simulink model "exp2_model"  (R2019b)
settings: Solver=FixedStepAuto  StartTime=0.0  StopTime=5  FixedStep=0.000001  RelTol=1e-3
values from neighbouring files (symbols this model uses):
  Io = 0    [exp2_script.m]
  Jeq = 1.16e-6+.5*0.068*.0248^2    (= 2.207136e-05)    [exp2_script.m]
  K = 1/(km+Rm*Io)    (= 19.9203187251)    [exp2_script.m]    (also in measured_data_plots.m = 14.5)
  km = 0.0502    [exp2_script.m]
  kt = 0.0502    [exp2_script.m]
  Ktd = -Rm/(kt*km+Rm*kt*Io)    (= -4206.28243996)    [exp2_script.m]
  Rm = 10.6    [exp2_script.m]
  Rm_measured = 1/ft.p1    [resistance_measurements.m]
  tau = Jeq*Rm/(kt*km+Rm*kt*Io)    (= 0.0928383739941)    [exp2_script.m]    (also in measured_data_plots.m = 0.09)
  tau_td = Jeq*Rm/(kt*km+Rm*kt*Io)    (= 0.0928383739941)    [exp2_script.m]
  wf = 1/0.1    (= 10)    [exp2_script.m]
undefined symbols (not defined in the file or in its folder): ki, kp
libraries: simulink x1, powerlib_meascontrol x1
settings Model: SimulationMode=accelerator  Creator=irex  LastModifiedBy=isaac
settings SolverCC: AlgebraicLoopSolver=LineSearch
settings SFSimCC: CustomCodeUndefinedFunction=UseInterfaceOnly

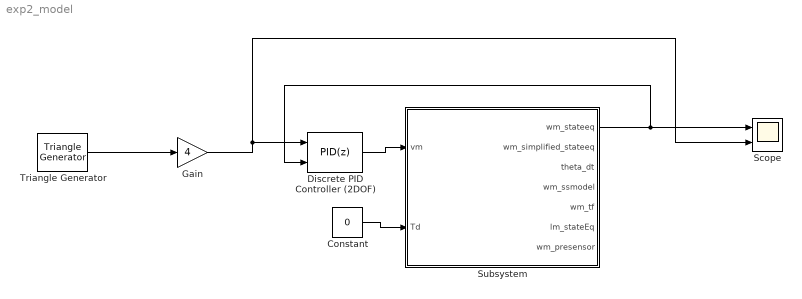
== system exp2_model ==
  Constant : Constant  Value=0
  Discrete PID Controller (2DOF) : simulink/Continuous/PID Controller (2DOF)  Controller=PID  Form=Parallel  TimeDomain=Discrete-time  SampleTime=-1  IntegratorMethod=Forward Euler  FilterMethod=Forward Euler  ControllerParametersSource=internal  P=kp  I=ki  D=0  UseFilter=on  N=100  b=1  c=1  TunerSelectOption=Transfer Function Based (PID Tuner App)  InitialConditionSource=internal  InitialConditionForIntegrator=0  InitialConditionForFilter=0  DifferentiatorICPrevScaledInput=0  ExternalReset=none  TrackingMode=off  Kt=1  LimitOutput=off  UpperSaturationLimit=inf  LowerSaturationLimit=-inf  LinearizeAsGain=off  AntiWindupMode=none  Kb=1  POutMin=[]  POutMax=[]  IOutMin=[]  IOutMax=[]  DOutMin=[]  DOutMax=[]  NOutMin=[]  NOutMax=[]  bOutMin=[]  bOutMax=[]  cOutMin=[]  cOutMax=[]  SumOutMin=[]  SumOutMax=[]  SaturationOutMin=[]  SaturationOutMax=[]  PParamMin=[]  PParamMax=[]  IParamMin=[]  IParamMax=[]  DParamMin=[]  DParamMax=[]  NParamMin=[]  NParamMax=[]  bParamMin=[]  bParamMax=[]  cParamMin=[]  cParamMax=[]  KbParamMin=[]  KbParamMax=[]  KtParamMin=[]  KtParamMax=[]  KbOutMin=[]  KbOutMax=[]  KtOutMin=[]  KtOutMax=[]  IntegratorOutMin=[]  IntegratorOutMax=[]  FilterOutMin=[]  FilterOutMax=[]  SumI1OutMin=[]  SumI1OutMax=[]  SumI2OutMin=[]  SumI2OutMax=[]  SumI3OutMin=[]  SumI3OutMax=[]  SumI4OutMin=[]  SumI4OutMax=[]  SumDOutMin=[]  SumDOutMax=[]  Sum1OutMin=[]  Sum1OutMax=[]  Sum2OutMin=[]  Sum2OutMax=[]  Sum3OutMin=[]  Sum3OutMax=[]  DifferentiatorOutMin=[]  DifferentiatorOutMax=[]  FilterDiffOutCoefMin=[]  FilterDiffOutCoefMax=[]  ReciprocalOutMin=[]  ReciprocalOutMax=[]  SumDenOutMin=[]  SumDenOutMax=[]  SumNumOutMin=[]  SumNumOutMax=[]  DivideOutMin=[]  DivideOutMax=[]  IntegratorContinuousStateAttributes=''  IntegratorStateMustResolveToSignalObject=off  IntegratorRTWStateStorageClass=Auto  FilterContinuousStateAttributes=''  FilterStateMustResolveToSignalObject=off  FilterRTWStateStorageClass=Auto  ParallelPVariant=InternalParameters  IdealPVariant=Disabled  IVariant=InternalParameters  DVariant=InternalParameters  bVariant=InternalParameters  cVariant=InternalParameters  IntegratorVariant=Discrete  SatVariant=Disabled  AWVariant=Passthrough  PCopyVariant=Disabled  TRVariant=Disabled  FdbkBlocksVariant=Forward  IdealPFdbkVariant=Disabled  SatFdbkVariant=Disabled  DerivativeFilterVariant=ForwardEulerFilter  NVariant=InternalParameters  NCopyVariant=Disabled  FilterICVariant=InternalICsFilter  IntegratorICVariant=InternalICs  ExternalResetVariant=Disabled  TRSumVariant=Passthrough  SumFdbkVariant=Disabled  SumVariant=Sum_PID
  Gain : Gain  Gain=4
  Scope : Scope  NumInputPorts=2
  Subsystem : Subsystem
  Triangle Generator : powerlib_meascontrol/Pulse & Signal Generators/Triangle Generator  Freq=1  Phase=90  Ts=0
      settings: SourceProductName=Simscape Electrical
  wires:
  Subsystem/1(wm_stateeq) -> Discrete PID Controller (2DOF)/2, Scope/1
  Constant/1 -> Subsystem/2(Td)
  Triangle Generator/1 -> Gain/1
  Gain/1 -> Discrete PID Controller (2DOF)/1, Scope/2
  Discrete PID Controller (2DOF)/1 -> Subsystem/1(vm)

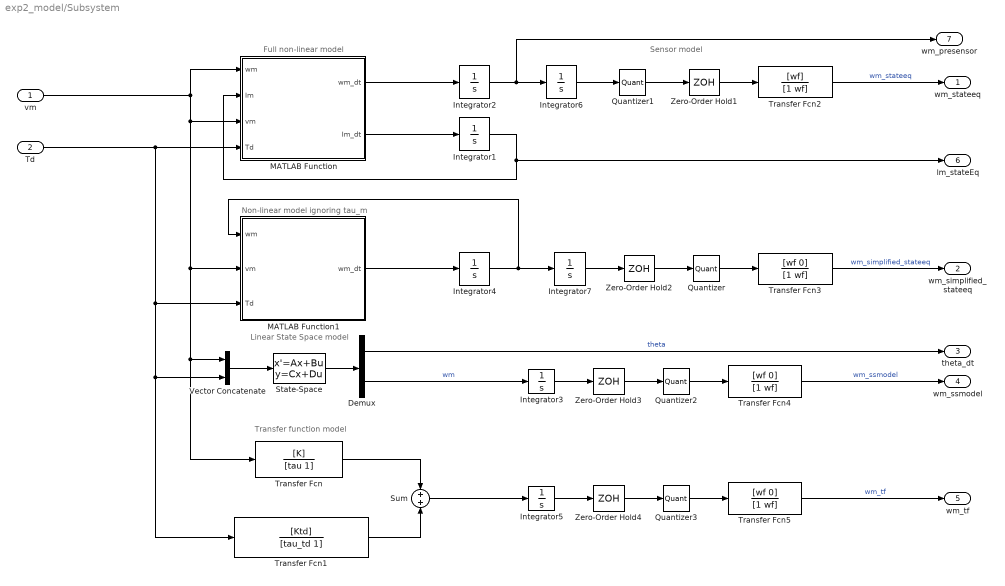
== system exp2_model/Subsystem ==
  note: Sensor model
  note: Transfer function model
  note: Linear State Space model
  note: Non-linear model ignoring tau_m
  note: Full non-linear model
  vm : Inport
  Td : Inport  Port=2
  Demux : Demux  Outputs=2
  Integrator{1..7} (7 alike) : Integrator
  MATLAB Function : MATLAB Function  TreatAsAtomicUnit=on
  MATLAB Function1 : MATLAB Function  TreatAsAtomicUnit=on
  Quantizer : Quantizer  QuantizationInterval=0.00153336666666666666666666666667
  Quantizer1 : Quantizer  QuantizationInterval=1/1024
  Quantizer2 : Quantizer  QuantizationInterval=0.00153336666666666666666666666667
  Quantizer3 : Quantizer  QuantizationInterval=0.00153336666666666666666666666667
  State-Space : StateSpace  A=[0 1; 0 -(km*kt+Rm*kt*Io)/(Jeq*Rm_measured)]  B=[0 0; kt/(Jeq*Rm_measured) -1/Jeq]  C=[1 0; 0 1]  D=[0 0; 0 0]  InitialCondition=0
  Sum : Sum  Inputs=+|+
  Transfer Fcn : TransferFcn  Numerator=[K]  Denominator=[tau 1]
  Transfer Fcn1 : TransferFcn  Numerator=[Ktd]  Denominator=[tau_td 1]
  Transfer Fcn2 : TransferFcn  Numerator=[wf]  Denominator=[1 wf]
  Transfer Fcn3 : TransferFcn  Numerator=[wf 0]  Denominator=[1 wf]
  Transfer Fcn4 : TransferFcn  Numerator=[wf 0]  Denominator=[1 wf]
  Transfer Fcn5 : TransferFcn  Numerator=[wf 0]  Denominator=[1 wf]
  Vector Concatenate : Concatenate
  Zero-Order Hold{1..4} (4 alike) : ZeroOrderHold  SampleTime=.01
  wm_stateeq : Outport
  wm_simplified_stateeq : Outport  Port=2
  theta_dt : Outport  Port=3
  wm_ssmodel : Outport  Port=4
  wm_tf : Outport  Port=5
  lm_stateEq : Outport  Port=6
  wm_presensor : Outport  Port=7
  wires:
  Transfer Fcn4/1 -> wm_ssmodel/1  "wm_ssmodel"
  Transfer Fcn3/1 -> wm_simplified_stateeq/1  "wm_simplified_stateeq"
  Integrator3/1 -> Zero-Order Hold3/1
  Demux/1 -> theta_dt/1  "theta"
  Integrator5/1 -> Zero-Order Hold4/1
  Quantizer2/1 -> Transfer Fcn4/1
  State-Space/1 -> Demux/1
  Zero-Order Hold4/1 -> Quantizer3/1
  MATLAB Function/1(wm_dt) -> Integrator2/1
  Quantizer/1 -> Transfer Fcn3/1
  Quantizer3/1 -> Transfer Fcn5/1
  Zero-Order Hold2/1 -> Quantizer/1
  Integrator7/1 -> Zero-Order Hold2/1
  Td/1 -> MATLAB Function1/3(Td), Transfer Fcn1/1, Vector Concatenate/2, MATLAB Function/4(Td)
  MATLAB Function1/1(wm_dt) -> Integrator4/1
  Integrator4/1 -> MATLAB Function1/1(wm), Integrator7/1
  Vector Concatenate/1 -> State-Space/1
  Sum/1 -> Integrator5/1
  Transfer Fcn5/1 -> wm_tf/1  "wm_tf"
  Transfer Fcn1/1 -> Sum/2
  MATLAB Function/2(Im_dt) -> Integrator1/1
  Transfer Fcn/1 -> Sum/1
  Integrator1/1 -> lm_stateEq/1, MATLAB Function/2(Im)
  vm/1 -> MATLAB Function/1(wm), Transfer Fcn/1, Vector Concatenate/1, MATLAB Function1/2(vm), MATLAB Function/3(vm)
  Demux/2 -> Integrator3/1  "wm"
  Zero-Order Hold3/1 -> Quantizer2/1
  Integrator2/1 -> wm_presensor/1, Integrator6/1
  Quantizer1/1 -> Zero-Order Hold1/1
  Zero-Order Hold1/1 -> Transfer Fcn2/1
  Integrator6/1 -> Quantizer1/1
  Transfer Fcn2/1 -> wm_stateeq/1  "wm_stateeq"

== matlab function exp2_model/Subsystem/MATLAB Function1 ==
  data: wm input; wm_dt output; vm input; Td input
function wm_dt  = wmStateEq_simplified(wm, vm, Td)
    if abs(vm) >= 15 
        vm = 15 * sign(vm);
    end
    
    Jeq = 1.16e-6+.5*0.068*.0248^2;
    kt = 0.0575;
    Io = .0471;
    I1 = 3.7e-5;
    I2 = 6.2e-8;
%     Io = 0;
%     I1 = 0;
%     I2 = 0;
    Rm = 10.9;
    km = kt;
    tau_m = 0;
    
    Im = (vm - km*wm*(1+tau_m))/Rm;
    
    wm_dt = 1/Jeq * (kt * (Im - Io*sign(wm) - I1*wm - I2*wm^2) - Td);
end

== matlab function exp2_model/Subsystem/MATLAB Function ==
  data: wm input; wm_dt output; Im input; Im_dt output; vm input; Td input
function [wm_dt, Im_dt] = wmStateEq(wm, Im, vm, Td)
    if abs(vm) >= 15
        vm = 15 * sign(vm);
    end
    if abs(Im) > 1.5
        Im = 1.5;
    end
    
    Jeq = 1.16e-6+.5*0.068*.0248^2;
    kt = 0.0575;
    Io = .0471;
    I1 = 3.7e-5;
    I2 = 6.2e-8;
%     Io = 0;
%     I1 = 0;
%     I2 = 0;
    Rm = 10.9;
    km = kt;
    tau_m = 8.8e-05;
    L = 0.82e-3;
    
    wm_dt = 1/Jeq * (kt * (Im - Io*sign(wm) - I1*wm - I2*wm^2) - Td);
    Im_dt = 1/L * (vm - Im*Rm - km * wm * (1 + tau_m*wm));
end
